simulink model "Experiment1"  (R2025b)
settings: Solver=ode4  StartTime=0.0  StopTime=tsim  FixedStep=baseRate  RelTol=1e-6  AbsTol=1e-6
values from neighbouring files (symbols this model uses):
  a1 = 0.1933    [fmincon_solver_v50.m]    (also in fmincon_solver_v51.m; fmincon_solver_v65_ultrafast.m)
  a2 = 0.1933    [fmincon_solver_v50.m]    (also in fmincon_solver_v51.m; fmincon_solver_v65_ultrafast.m)
  a3 = 0.0621    [fmincon_solver_v50.m]    (also in fmincon_solver_v51.m; fmincon_solver_v65_ultrafast.m)
  b0 = 0.2304    [fmincon_solver_v50.m]    (also in fmincon_solver_v51.m; fmincon_solver_v65_ultrafast.m)
  b1 = 0.1117    [fmincon_solver_v50.m]    (also in fmincon_solver_v51.m; fmincon_solver_v65_ultrafast.m)
  b2 = 0.1057    [fmincon_solver_v50.m]    (also in fmincon_solver_v51.m; fmincon_solver_v65_ultrafast.m)
  b3 = 0.0159    [fmincon_solver_v50.m]    (also in fmincon_solver_v51.m; fmincon_solver_v65_ultrafast.m)
  Gamma1_el = 0.12    [Run_Initializer.m]
  Gamma1_sh = 0.005    [Run_Initializer.m]
  Gamma1_wr = 0.025    [Run_Initializer.m]
  Gamma2_el = 5    [Run_Initializer.m]
  Gamma2_sh = 5    [Run_Initializer.m]
  Gamma2_wr = 5    [Run_Initializer.m]
  Gamma3_el = 10    [Run_Initializer.m]
  Gamma3_sh = 40    [Run_Initializer.m]
  Gamma3_wr = 40    [Run_Initializer.m]
  Gamma4_el = 0.039    [Run_Initializer.m]
  Gamma4_sh = 0.015    [Run_Initializer.m]
  Gamma4_wr = 0.029    [Run_Initializer.m]
  Gamma5_el = 800    [Run_Initializer.m]
  Gamma5_sh = 800    [Run_Initializer.m]
  Gamma5_wr = 800    [Run_Initializer.m]
  Gamma6_el = 0.000001    (= 1e-06)    [Run_Initializer.m]
  Gamma6_sh = 0.005    [Run_Initializer.m]
  Gamma6_wr = 0.02    [Run_Initializer.m]
  Kd_elarm = 0.8    [Run_Initializer.m]
  Kd_sharm = 1.0    (= 1)    [Run_Initializer.m]
  Kd_wrarm = 0.6    [Run_Initializer.m]
  Kp_elarm = 1.2    [Run_Initializer.m]
  Kp_sharm = 1.5    [Run_Initializer.m]
  Kp_wrarm = 1.0    (= 1)    [Run_Initializer.m]
  PWMFreq = 5    [Run_Initializer.m]
  Tz_lim_elarm = .1    (= 0.1)    [Run_Initializer.m]
  Tz_lim_sharm = .1    (= 0.1)    [Run_Initializer.m]
  Tz_lim_wrarm = .1    (= 0.1)    [Run_Initializer.m]
undefined symbols (not defined in the file or in its folder): baseRate, dataRate, DiscIntNeverNeededParam, drop_states_ARM, drop_states_BLACK, drop_states_BLUE, drop_states_RED, F_red_X_nominal, F_red_Y_nominal, F_thrusters_BLACK, F_thrusters_BLUE, F_thrusters_RED, home_states_BLACK, home_states_BLUE, home_states_RED, IBLACK, IBLUE, IDIST, IEE, init_states_BLACK, init_states_BLUE, init_states_RED, IPROX, IRED, K_BLACK, K_BLUE, K_RED, Kd_tb, Kd_tblue, Kd_tr, Kd_xb, Kd_xblue, Kd_xr, Kd_yb, Kd_yblue, Kd_yr, Kp_tb, Kp_tblue, Kp_tr, Kp_xb, Kp_xblue, Kp_xr, Kp_yb, Kp_yblue, Kp_yr, mBLACK, mBLUE, mDIST, mEE, mPROX, mRED, Phase0_End, Phase1_End, Phase2_End, Phase3_End, Phase3_SubPhase1_End, Phase3_SubPhase2_End, Phase3_SubPhase3_End, Phase3_SubPhase4_End, Phase4_End ... (+10)
libraries: simulink x30, nvidiaSharedBlocks x19, MainLibrary x6, dspinverses x3, nvidiaIMUSensorslib x1
(part 7 of 8)

== system Experiment1/Simulate Plant Dynamics/RED and ARM Dynamics/RED + ARM/Calculated & Store Measured States/Subsystem3/Enabled Subsystem ==
  y : Inport
  dt : Inport  Port=2
  Enable : EnablePort
  Constant2 : Constant  Value=0.1
  Delay : Delay  DelayLength=1
  MATLAB Function : MATLAB Function  TreatAsAtomicUnit=on
  dy/dt : Outport
  wires:
  Constant2/1 -> MATLAB Function/3(tau)
  dt/1 -> MATLAB Function/2(dt)
  Delay/1 -> MATLAB Function/4(ema_prev)
  MATLAB Function/2(ema) -> Delay/1
  y/1 -> MATLAB Function/1(y)
  MATLAB Function/1(dy) -> dy/dt/1

== system Experiment1/Simulate Plant Dynamics/RED and ARM Dynamics/RED + ARM/Calculated & Store Measured States/Subsystem4/Enabled Subsystem ==
  y : Inport
  dt : Inport  Port=2
  Enable : EnablePort
  Constant2 : Constant  Value=0.1
  Delay : Delay  DelayLength=1
  MATLAB Function : MATLAB Function  TreatAsAtomicUnit=on
  dy/dt : Outport
  wires:
  Constant2/1 -> MATLAB Function/3(tau)
  dt/1 -> MATLAB Function/2(dt)
  Delay/1 -> MATLAB Function/4(ema_prev)
  MATLAB Function/2(ema) -> Delay/1
  y/1 -> MATLAB Function/1(y)
  MATLAB Function/1(dy) -> dy/dt/1

== system Experiment1/Simulate Plant Dynamics/RED and ARM Dynamics/RED + ARM/Calculated & Store Measured States/Subsystem5/Enabled Subsystem ==
  y : Inport
  dt : Inport  Port=2
  Enable : EnablePort
  Constant2 : Constant  Value=0.1
  Delay : Delay  DelayLength=1
  MATLAB Function : MATLAB Function  TreatAsAtomicUnit=on
  dy/dt : Outport
  wires:
  Constant2/1 -> MATLAB Function/3(tau)
  dt/1 -> MATLAB Function/2(dt)
  Delay/1 -> MATLAB Function/4(ema_prev)
  MATLAB Function/2(ema) -> Delay/1
  y/1 -> MATLAB Function/1(y)
  MATLAB Function/1(dy) -> dy/dt/1

== system Experiment1/Simulate Plant Dynamics/RED and ARM Dynamics/RED + ARM/Data @ Measurement Rate/Calculate True Time Step/Enabled Subsystem3 ==
  y2-y1 : Inport
  Enable : EnablePort
  dy(t)/dt : Outport
  wires:
  y2-y1/1 -> dy(t)/dt/1

== system Experiment1/Simulate Plant Dynamics/RED and ARM Dynamics/RED Only/Calculated & Store Measured States/Subsystem1/Enabled Subsystem ==
  y : Inport
  dt : Inport  Port=2
  Enable : EnablePort
  Constant2 : Constant  Value=0.1
  Delay : Delay  DelayLength=1
  MATLAB Function : MATLAB Function  TreatAsAtomicUnit=on
  dy/dt : Outport
  wires:
  Constant2/1 -> MATLAB Function/3(tau)
  dt/1 -> MATLAB Function/2(dt)
  Delay/1 -> MATLAB Function/4(ema_prev)
  MATLAB Function/2(ema) -> Delay/1
  y/1 -> MATLAB Function/1(y)
  MATLAB Function/1(dy) -> dy/dt/1

== system Experiment1/Simulate Plant Dynamics/RED and ARM Dynamics/RED Only/Calculated & Store Measured States/Subsystem2/Enabled Subsystem ==
  y : Inport
  dt : Inport  Port=2
  Enable : EnablePort
  Constant2 : Constant  Value=0.1
  Delay : Delay  DelayLength=1
  MATLAB Function : MATLAB Function  TreatAsAtomicUnit=on
  dy/dt : Outport
  wires:
  Constant2/1 -> MATLAB Function/3(tau)
  dt/1 -> MATLAB Function/2(dt)
  Delay/1 -> MATLAB Function/4(ema_prev)
  MATLAB Function/2(ema) -> Delay/1
  y/1 -> MATLAB Function/1(y)
  MATLAB Function/1(dy) -> dy/dt/1

== system Experiment1/Simulate Plant Dynamics/RED and ARM Dynamics/RED Only/Data @ Measurement Rate/Calculate True Time Step/Enabled Subsystem3 ==
  y2-y1 : Inport
  Enable : EnablePort
  dy(t)/dt : Outport
  wires:
  y2-y1/1 -> dy(t)/dt/1

== matlab function Experiment1/3 - Control/Default LQR Control (BLUE)/Calculate Error/MATLAB Function ==
  data: Rz_path input; Rz_error output; Rz_measured input
function Rz_error = SmoothAngularDifference(Rz_path, Rz_measured)

    Rz_error = mod(Rz_measured-Rz_path+pi, 2*pi)-pi;


end

== matlab function Experiment1/3 - Control/Default PD Control (BLUE)/Calculate Error/MATLAB Function ==
  data: Rz_path input; Rz_error output; Rz_measured input
function Rz_error = SmoothAngularDifference(Rz_path, Rz_measured)

    Rz_error = mod(Rz_measured-Rz_path+pi, 2*pi)-pi;


end

== matlab function Experiment1/Simulate Plant Dynamics/RED and ARM Dynamics/RED + ARM/Calculated & Store Measured States/Subsystem3/Enabled Subsystem/MATLAB Function ==
  data: y input; dy output; dt input; tau input; ema_prev input; ema output
function [dy, ema] = realtime_derivative_ema(y, dt, tau, ema_prev)
    % Compute smoothed derivative using Exponential Moving Average
    %
    % Inputs:
    %   y        : Current measurement
    %   dt       : Time step
    %   tau      : Time constant for EMA filter (larger = more smoothing)
    %   ema_prev : Previous EMA value
    %
    % Outputs:
    %   dy  : Smoothed derivative estimate
    %   ema : Updated EMA value
    
    % Calculate smoothing factor from time constant
    alpha = 1 - exp(-dt ./ tau);
    
    % Update Exponential Moving Average
    ema = alpha .* y + (1 - alpha) .* ema_prev;
    
    % Compute derivative using finite difference on smoothed values
    dy = (ema - ema_prev) ./ dt;
end

== matlab function Experiment1/Simulate Plant Dynamics/RED and ARM Dynamics/RED Only/Calculated & Store Measured States/Subsystem2/Enabled Subsystem/MATLAB Function ==
  data: y input; dy output; dt input; tau input; ema_prev input; ema output
function [dy, ema] = realtime_derivative_ema(y, dt, tau, ema_prev)
    % Compute smoothed derivative using Exponential Moving Average
    %
    % Inputs:
    %   y        : Current measurement
    %   dt       : Time step
    %   tau      : Time constant for EMA filter (larger = more smoothing)
    %   ema_prev : Previous EMA value
    %
    % Outputs:
    %   dy  : Smoothed derivative estimate
    %   ema : Updated EMA value
    
    % Calculate smoothing factor from time constant
    alpha = 1 - exp(-dt ./ tau);
    
    % Update Exponential Moving Average
    ema = alpha .* y + (1 - alpha) .* ema_prev;
    
    % Compute derivative using finite difference on smoothed values
    dy = (ema - ema_prev) ./ dt;
end

== matlab function Experiment1/Simulate Plant Dynamics/BLACK Dynamics/Calculated & Store Measured States/Subsystem1/Enabled Subsystem/MATLAB Function ==
  data: y input; dy output; dt input; tau input; ema_prev input; ema output
function [dy, ema] = realtime_derivative_ema(y, dt, tau, ema_prev)
    % Compute smoothed derivative using Exponential Moving Average
    %
    % Inputs:
    %   y        : Current measurement
    %   dt       : Time step
    %   tau      : Time constant for EMA filter (larger = more smoothing)
    %   ema_prev : Previous EMA value
    %
    % Outputs:
    %   dy  : Smoothed derivative estimate
    %   ema : Updated EMA value
    
    % Calculate smoothing factor from time constant
    alpha = 1 - exp(-dt ./ tau);
    
    % Update Exponential Moving Average
    ema = alpha .* y + (1 - alpha) .* ema_prev;
    
    % Compute derivative using finite difference on smoothed values
    dy = (ema - ema_prev) ./ dt;
end

== matlab function Experiment1/Simulate Plant Dynamics/RED and ARM Dynamics/RED Only/Data @ Measurement Rate/Calculate True Time Step/MATLAB Function ==
  data: dt input; dt_out output; dataRate input
function dt_out = CheckforInvalidTime(dt, dataRate)

    if dt <= 0

        dt_out = dataRate;

    else

        dt_out = dt;

    end


end

== matlab function Experiment1/Thruster Control Code/Change BLACK Behavior/Calculate Duty Cycle/MATLAB Function5 ==
  data: H_final output; u_desired input; duty_cycles output; x0 input; thruster_dist2CG_RED parameter; F_red_X_nominal parameter; F_red_Y_nominal parameter; max_iters parameter; tol parameter
function [H_final, duty_cycles] = optimize_duty_cycle_with_decay( ...
    u_desired, x0, thruster_dist2CG_RED, F_red_X_nominal, F_red_Y_nominal, max_iters, tol)
    %OPTIMIZE_DUTY_CYCLE_WITH_DECAY 
    %   Iteratively optimizes thruster duty cycles while updating thrust decay.
    %
    %   Inputs:
    %       u_desired           - Desired force/torque vector [Fx; Fy; M] (3x1)
    %       x0                  - Initial guess for duty cycles (8x1)
    %       thruster_dist2CG_RED- Distances of thrusters from CG (vector, mm)
    %       F_red_X_nominal     - Nominal X-direction thruster force (scalar, N)
    %       F_red_Y_nominal     - Nominal Y-direction thruster force (scalar, N)
    %       max_iters           - Maximum optimization iterations
    %       tol                 - Convergence tolerance (on duty cycles)
    %
    %   Outputs:
    %       H_final     - Final H-matrix including thrust decay (3x8)
    %       duty_cycles - Optimized duty cycles (8x1)
    %

    % ---------------------------
    % Initialization
    % ---------------------------
    num_thrusters      = length(x0); %#ok<NASGU> % reserved if needed later
    duty_cycles        = x0;                     % current solution
    thrust_decay_factor = 1;                     % initial decay
    prev_duty_cycles   = duty_cycles + 2*tol;    % force first iteration

    % ---------------------------
    % Iterative optimization
    % ---------------------------
    for iter = 1:max_iters
        % Build system matrix H with current decay factor
        H = MakeHWithDecay(thruster_dist2CG_RED, F_red_X_nominal, ...
                           thrust_decay_factor, F_red_Y_nominal);

        % Solve constrained least squares (box constraints: 0 ≤ x ≤ 1)
        duty_cycles = custom_constrained_least_squares(H, u_desired, duty_cycles);

        % Update decay factor based on the current duty cycles
        [thrust_decay_factor, ~] = check_thrust_decay(duty_cycles);

        % Check convergence (∞-norm difference)
        if norm(duty_cycles - prev_duty_cycles, Inf) < tol
            H_final = MakeHWithDecayRecalculateForce(thruster_dist2CG_RED, ...
                        F_red_X_nominal, thrust_decay_factor, F_red_Y_nominal);
            return;
        end

        % Update reference for next iteration
        prev_duty_cycles = duty_cycles;
    end

    % If not converged within max_iters, return final H with last decay
    H_final = MakeHWithDecayRecalculateForce(thruster_dist2CG_RED, ...
                F_red_X_nominal, thrust_decay_factor, F_red_Y_nominal);
end


% ========================================================================
% Custom Constrained Least Squares Solver
% ========================================================================
function x_opt = custom_constrained_least_squares(H, b, x0)
    %CUSTOM_CONSTRAINED_LEAST_SQUARES
    %   Solves min_x ||H*x - b||^2 subject to 0 <= x <= 1
    %   using projected gradient descent with backtracking line search.
    %
    %   Inputs:
    %       H   - System matrix (3x8)
    %       b   - Desired vector (3x1)
    %       x0  - Initial guess (8x1)
    %
    %   Output:
    %       x_opt - Optimal duty cycle vector (8x1)

    % Parameters
    max_iterations = 100;
    tolerance      = 1e-6;
    alpha          = 0.01;  % initial step size
    beta           = 0.5;   % backtracking factor

    % Initialization
    x      = x0;
    x_prev = x0 + 2*tolerance;

    % Precompute matrices
    HtH = H' * H;
    Htb = H' * b;

    for iter = 1:max_iterations
        % Gradient of ||H*x - b||^2
        gradient = 2 * (HtH*x - Htb);

        % Store objective for comparison
        current_obj = norm(H*x - b)^2;

        % Backtracking line search
        step_size = alpha;
        for ls_iter = 1:20
            x_new = x - step_size * gradient;
            x_new = max(0, min(1, x_new)); % project into [0,1]

            new_obj = norm(H*x_new - b)^2;
            if new_obj < current_obj
                break; % accept step
            else
                step_size = step_size * beta;
            end
        end

        % Update
        x = x_new;

        % Convergence check
        if norm(x - x_prev) < tolerance
            break;
        end

        % Adaptive step size tuning
        if iter > 1 && new_obj < current_obj
            alpha = min(alpha * 1.1, 0.1); % speed up if progress
        else
            alpha = alpha * 0.9;           % slow down otherwise
        end

        % Store for next iteration
        x_prev = x;
    end

    x_opt = x;
end


% ========================================================================
% Construct H-matrix (with decay factor)
% ========================================================================
function H = MakeHWithDecay(thruster_dist2CG, F_X_nominal, thrust_decay_factor, F_Y_nominal)
    %MAKEHWITHDECAY
    %   Builds the H matrix that maps thruster duty cycles to [Fx; Fy; M],
    %   applying thrust decay.
    %
    %   Outputs H as (3x8)

    % Convert thruster arm distances to meters
    adjusted_dist = thruster_dist2CG / 1000;

    % Thruster directions (X, Y, and moment arm)
    Vec1 = [-1; -1;  0;  0;  1;  1;  0;  0]; % X
    Vec2 = [ 0;  0;  1;  1;  0;  0; -1; -1]; % Y
    Vec3 = adjusted_dist;                    % moment (Z)

    Mat1 = [Vec1, Vec2, Vec3]';

    % Thruster forces (scaled by decay)
    F_thrusters = [F_X_nominal; F_X_nominal; ...
                   F_Y_nominal; F_Y_nominal; ...
                   F_X_nominal; F_X_nominal; ...
                   F_Y_nominal; F_Y_nominal] * thrust_decay_factor;

    % Build diagonal scaling
    Mat2 = diag(F_thrusters / 2);

    % Final mapping
    H = Mat1 * Mat2;
end


% ========================================================================
% Construct H-matrix (recalculate full force with decay)
% ========================================================================
function H = MakeHWithDecayRecalculateForce(thruster_dist2CG, F_X_nominal, thrust_decay_factor, F_Y_nominal)
    %MAKEHWITHDECAYRECALCULATEFORCE
    %   Same as MakeHWithDecay but applies full nominal force scaling.

    adjusted_dist = thruster_dist2CG / 1000;

    Vec1 = [-1; -1;  0;  0;  1;  1;  0;  0];
    Vec2 = [ 0;  0;  1;  1;  0;  0; -1; -1];
    Vec3 = adjusted_dist;

    Mat1 = [Vec1, Vec2, Vec3]';

    F_thrusters = [F_X_nominal; F_X_nominal; ...
                   F_Y_nominal; F_Y_nominal; ...
                   F_X_nominal; F_X_nominal; ...
                   F_Y_nominal; F_Y_nominal] * thrust_decay_factor;

    Mat2 = diag(F_thrusters);

    H = Mat1 * Mat2;
end


% ========================================================================
% Thrust Decay Update Rule
% ========================================================================
function [thrust_decay_factor, count] = check_thrust_decay(PWMs)
    %CHECK_THRUST_DECAY
    %   Updates thrust decay factor based on average duty cycle.
    %
    %   Inputs:
    %       PWMs - Duty cycle vector (8x1)
    %
    %   Outputs:
    %       thrust_decay_factor - Adjusted decay factor (scalar)
    %       count               - Number of active thrusters

    % Normalize if needed
    if max(PWMs) > 1
        PWMs = PWMs / max(PWMs);
    end
    
    % Active thrusters
    count = sum(PWMs > 0);
    
    % Mean duty cycle (only active thrusters)
    avg_duty = sum(max(PWMs, 0)) / max(count, 1);
    
    % Update rule (piecewise)
    if avg_duty < 0.3 || count == 0
        thrust_decay_factor = 1;
    else
        thrust_decay_factor = max(0.6 - 2*avg_duty + 1, 0.5);
    end
end

== matlab function Experiment1/Simulate Plant Dynamics/RED and ARM Dynamics/RED + ARM/Calculated & Store Measured States/Subsystem4/Enabled Subsystem/MATLAB Function ==
  data: y input; dy output; dt input; tau input; ema_prev input; ema output
function [dy, ema] = realtime_derivative_ema(y, dt, tau, ema_prev)
    % Compute smoothed derivative using Exponential Moving Average
    %
    % Inputs:
    %   y        : Current measurement
    %   dt       : Time step
    %   tau      : Time constant for EMA filter (larger = more smoothing)
    %   ema_prev : Previous EMA value
    %
    % Outputs:
    %   dy  : Smoothed derivative estimate
    %   ema : Updated EMA value
    
    % Calculate smoothing factor from time constant
    alpha = 1 - exp(-dt ./ tau);
    
    % Update Exponential Moving Average
    ema = alpha .* y + (1 - alpha) .* ema_prev;
    
    % Compute derivative using finite difference on smoothed values
    dy = (ema - ema_prev) ./ dt;
end

== matlab function Experiment1/PhaseSpace Camera Code/Use Hardware to Obtain States/Store RED Data/Subsystem1/Enabled Subsystem/MATLAB Function ==
  data: y input; dy output; dt input; tau input; ema_prev input; ema output
function [dy, ema] = realtime_derivative_ema(y, dt, tau, ema_prev)
    % Compute smoothed derivative using Exponential Moving Average
    %
    % Inputs:
    %   y        : Current measurement
    %   dt       : Time step
    %   tau      : Time constant for EMA filter (larger = more smoothing)
    %   ema_prev : Previous EMA value
    %
    % Outputs:
    %   dy  : Smoothed derivative estimate
    %   ema : Updated EMA value
    
    % Calculate smoothing factor from time constant
    alpha = 1 - exp(-dt ./ tau);
    
    % Update Exponential Moving Average
    ema = alpha .* y + (1 - alpha) .* ema_prev;
    
    % Compute derivative using finite difference on smoothed values
    dy = (ema - ema_prev) ./ dt;
end

== matlab function Experiment1/Simulate Plant Dynamics/BLACK Dynamics/Calculated & Store Measured States/Subsystem2/Enabled Subsystem/MATLAB Function ==
  data: y input; dy output; dt input; tau input; ema_prev input; ema output
function [dy, ema] = realtime_derivative_ema(y, dt, tau, ema_prev)
    % Compute smoothed derivative using Exponential Moving Average
    %
    % Inputs:
    %   y        : Current measurement
    %   dt       : Time step
    %   tau      : Time constant for EMA filter (larger = more smoothing)
    %   ema_prev : Previous EMA value
    %
    % Outputs:
    %   dy  : Smoothed derivative estimate
    %   ema : Updated EMA value
    
    % Calculate smoothing factor from time constant
    alpha = 1 - exp(-dt ./ tau);
    
    % Update Exponential Moving Average
    ema = alpha .* y + (1 - alpha) .* ema_prev;
    
    % Compute derivative using finite difference on smoothed values
    dy = (ema - ema_prev) ./ dt;
end

== matlab function Experiment1/Simulate Plant Dynamics/RED and ARM Dynamics/RED + ARM/Coriolis Function1 ==
  data: a1 parameter; a2 parameter; a3 parameter; b0 parameter; b1 parameter; b2 parameter; mPROX parameter; mDIST parameter; mEE parameter; Phi parameter; CoriolisS output; x input
function CoriolisS = CoriolisFunc3LINK(a1,a2,a3,b0,b1,b2,mPROX,mDIST,mEE,Phi,x)
%CORIOLISFUNC3LINK
%    CORIOLISS = CORIOLISFUNC3LINK(A1,A2,A3,B0,B1,B2,mPROX,mDIST,mEE,PHI,Q0,Q1,Q2,Q3,Q0_DOT,Q1_DOT,Q2_DOT,Q3_DOT)

%    This function was generated by the Symbolic Math Toolbox version 8.0.
%    05-Nov-2017 11:48:44

q0 = x(3);
q1 = x(4);
q2 = x(5);
q3 = x(6);

q0_dot = x(9);
q1_dot = x(10);
q2_dot = x(11);
q3_dot = x(12);

t2 = a1+b1;
t3 = a1.*mPROX;
t4 = mDIST.*t2;
t5 = mEE.*t2;
t6 = t3+t4+t5;
t7 = a2.*mDIST;
t8 = a2+b2;
t9 = mEE.*t8;
t10 = t7+t9;
t11 = pi.*(1.0./2.0);
t12 = q0_dot.*t6;
t13 = q1_dot.*t6;
t14 = q0+q1+t11;
t15 = cos(t14);
t16 = t12+t13;
t17 = q0_dot.*t10;
t18 = q1_dot.*t10;
t19 = q2_dot.*t10;
t20 = q0+q1+q2+t11;
t21 = cos(t20);
t22 = t17+t18+t19;
t23 = a3.*mEE.*q0_dot;
t24 = a3.*mEE.*q1_dot;
t25 = a3.*mEE.*q2_dot;
t26 = a3.*mEE.*q3_dot;
t27 = q0+q1+q2+q3+t11;
t28 = cos(t27);
t29 = t23+t24+t25+t26;
t30 = b0.*mPROX;
t31 = b0.*mDIST;
t32 = b0.*mEE;
t33 = t30+t31+t32;
t34 = (pi/2-Phi)+q0;
t35 = sin(t14);
t36 = sin(t20);
t37 = sin(t27);
t38 = q0_dot+q1_dot+q2_dot+q3_dot;
t39 = q0+q1+q2+q3;
t40 = a1.*b0.*mPROX.*q1_dot;
t41 = a1.*b0.*mDIST.*q1_dot;
t42 = a1.*b0.*mEE.*q1_dot;
t43 = b0.*b1.*mDIST.*q1_dot;
t44 = b0.*b1.*mEE.*q1_dot;
t45 = (pi/2-Phi)-q1;
t46 = cos(t45);
t47 = a2.*b0.*mDIST.*q1_dot;
t48 = a2.*b0.*mDIST.*q2_dot;
t49 = a2.*b0.*mEE.*q1_dot;
t50 = a2.*b0.*mEE.*q2_dot;
t51 = b0.*b2.*mEE.*q1_dot;
t52 = b0.*b2.*mEE.*q2_dot;
t53 = -(pi/2-Phi)+q1+q2;
t54 = cos(t53);
t55 = a3.*b0.*mEE.*q1_dot;
t56 = a3.*b0.*mEE.*q2_dot;
t57 = a3.*b0.*mEE.*q3_dot;
t58 = -(pi/2-Phi)+q1+q2+q3;
t59 = cos(t58);
t60 = a2.*b1.*mDIST.*q2_dot;
t61 = a1.*b2.*mEE.*q2_dot;
t62 = a2.*b1.*mEE.*q2_dot;
t63 = b1.*b2.*mEE.*q2_dot;
t64 = a1.*a2.*mDIST.*q2_dot;
t65 = a1.*a2.*mEE.*q2_dot;
t66 = sin(q2);
t67 = t60+t61+t62+t63+t64+t65;
t68 = a3.*b2.*mEE.*q3_dot;
t69 = a2.*a3.*mEE.*q3_dot;
t70 = sin(q3);
t71 = t68+t69;
t72 = a3.*b1.*mEE.*q2_dot;
t73 = a3.*b1.*mEE.*q3_dot;
t74 = a1.*a3.*mEE.*q2_dot;
t75 = a1.*a3.*mEE.*q3_dot;
t76 = q2+q3;
t77 = sin(t76);
t78 = t72+t73+t74+t75;
t79 = a2.*b0.*mDIST.*q0_dot;
t80 = a2.*b0.*mEE.*q0_dot;
t81 = b0.*b2.*mEE.*q0_dot;
t82 = t47+t48+t49+t50+t51+t52+t79+t80+t81;
t83 = a3.*b0.*mEE.*q0_dot;
t84 = t55+t56+t57+t83;
t85 = a1.*b0.*mPROX.*q0_dot;
t86 = a1.*b0.*mDIST.*q0_dot;
t87 = a1.*b0.*mEE.*q0_dot;
t88 = b0.*b1.*mDIST.*q0_dot;
t89 = b0.*b1.*mEE.*q0_dot;
t90 = a2.*b1.*mDIST.*q0_dot;
t91 = a1.*b2.*mEE.*q0_dot;
t92 = a2.*b1.*mDIST.*q1_dot;
t93 = a2.*b1.*mEE.*q0_dot;
t94 = a1.*b2.*mEE.*q1_dot;
t95 = a2.*b1.*mEE.*q1_dot;
t96 = b1.*b2.*mEE.*q0_dot;
t97 = b1.*b2.*mEE.*q1_dot;
t98 = a1.*a2.*mDIST.*q0_dot;
t99 = a1.*a2.*mDIST.*q1_dot;
t100 = a1.*a2.*mEE.*q0_dot;
t101 = a1.*a2.*mEE.*q1_dot;
t102 = t60+t61+t62+t63+t64+t65+t90+t91+t92+t93+t94+t95+t96+t97+t98+t99+t100+t101;
t103 = a3.*b1.*mEE.*q0_dot;
t104 = a3.*b1.*mEE.*q1_dot;
t105 = a1.*a3.*mEE.*q0_dot;
t106 = a1.*a3.*mEE.*q1_dot;
t107 = t72+t73+t74+t75+t103+t104+t105+t106;
t108 = t79+t80+t81;
t109 = t54.*t108;
t110 = t59.*t83;
t111 = t90+t91+t92+t93+t94+t95+t96+t97+t98+t99+t100+t101;
t112 = t66.*t111;
t113 = t103+t104+t105+t106;
t114 = t77.*t113;
t115 = a2.*q0_dot;
t116 = a2.*q1_dot;
t117 = a2.*q2_dot;
t118 = b2.*q0_dot;
t119 = b2.*q1_dot;
t120 = b2.*q2_dot;
t121 = t115+t116+t117+t118+t119+t120;
t122 = a3.*mEE.*t70.*t121;
t123 = a1.*q0_dot;
t124 = a1.*q1_dot;
t125 = b1.*q0_dot;
t126 = b1.*q1_dot;
t127 = t123+t124+t125+t126;
t128 = a3.*mEE.*t77.*t127;
CoriolisS = reshape([0.0,0.0,0.0,0.0,0.0,0.0,0.0,0.0,0.0,0.0,0.0,0.0,-t15.*t16-t21.*t22-t28.*t29-q0_dot.*t33.*cos(t34),-t16.*t35-t22.*t36-t29.*t37-q0_dot.*t33.*sin(t34),-t66.*t67-t70.*t71-t77.*t78-t46.*(t40+t41+t42+t43+t44)-t59.*(t55+t56+t57)-t54.*(t47+t48+t49+t50+t51+t52),t109+t110-t66.*t67-t70.*t71-t77.*t78+t46.*(t85+t86+t87+t88+t89),t109+t110+t112+t114-t70.*t71,t110+t122+t128,-t15.*t16-t21.*t22-t28.*t29,-t16.*t35-t22.*t36-t29.*t37,-t66.*t67-t54.*t82-t70.*t71-t59.*t84-t77.*t78-t46.*(t40+t41+t42+t43+t44+t85+t86+t87+t88+t89),-t66.*t67-t70.*t71-t77.*t78,t112+t114-t70.*t71,t122+t128,-t21.*t22-t28.*t29,-t22.*t36-t29.*t37,-t54.*t82-t70.*t71-t59.*t84-t66.*t102-t77.*t107,-t70.*t71-t66.*t102-t77.*t107,-a3.*mEE.*q3_dot.*t8.*t70,a3.*mEE.*t8.*t70.*(q0_dot+q1_dot+q2_dot),a3.*mEE.*t38.*sin(t39),-a3.*mEE.*t38.*cos(t39),-a3.*b0.*mEE.*t38.*t59-a3.*mEE.*t8.*t38.*t70-a3.*mEE.*t2.*t38.*t77,-a3.*mEE.*t8.*t38.*t70-a3.*mEE.*t2.*t38.*t77,-a3.*mEE.*t8.*t38.*t70,0.0],[6,6]);
end

== matlab function Experiment1/Simulate Plant Dynamics/BLACK Dynamics/Data @ Measurement Rate/Calculate True Time Step/MATLAB Function ==
  data: dt input; dt_out output; dataRate input
function dt_out = CheckforInvalidTime(dt, dataRate)

    if dt <= 0

        dt_out = dataRate;

    else

        dt_out = dt;

    end


end

== matlab function Experiment1/Simulate Plant Dynamics/RED and ARM Dynamics/RED + ARM/Inertia Function 1 ==
  data: mRED parameter; IRED parameter; Phi parameter; b0 parameter; a1 parameter; b1 parameter; a2 parameter; b2 parameter; a3 parameter; b3 parameter; mPROX parameter; mDIST parameter; mEE parameter; IPROX parameter; IDIST parameter; InertiaS output; x input; IEE parameter
function InertiaS = InertiaFunc3LINK(mRED, IRED, Phi, b0, a1, b1, a2, b2, a3, b3, mPROX, mDIST, mEE, IPROX, IDIST, x, IEE)

    q0 = x(3);
    q1 = x(4);
    q2 = x(5);
    q3 = x(6);
    
    t2 = a1+b1;
    t3 = a1.*mPROX;
    t4 = mDIST.*t2;
    t5 = mEE.*t2;
    t6 = q0+q1;
    t7 = cos(t6);
    t8 = t3+t4+t5;
    t9 = a2.*mDIST;
    t10 = a2+b2;
    t11 = mEE.*t10;
    t12 = q0+q1+q2;
    t13 = cos(t12);
    t14 = t9+t11;
    t15 = q0+q1+q2+q3;
    t16 = cos(t15);
    t17 = mRED+mPROX+mDIST+mEE;
    t18 = b0.*mPROX;
    t19 = b0.*mDIST;
    t20 = b0.*mEE;
    t21 = t18+t19+t20;
    t22 = (pi/2-Phi)+q0;
    t23 = sin(t6);
    t24 = sin(t12);
    t25 = sin(t15);
    t26 = a2.*mEE;
    t27 = b2.*mEE;
    t28 = t9+t26+t27;
    t29 = sin(t22);
    t86 = t7.*t8;
    t87 = t13.*t14;
    t88 = a3.*mEE.*t16;
    t30 = -t86-t87-t88-t21.*t29;
    t31 = cos(t22);
    t32 = t21.*t31;
    t89 = t8.*t23;
    t90 = t14.*t24;
    t91 = a3.*mEE.*t25;
    t33 = t32-t89-t90-t91;
    t34 = a1.^2;
    t35 = a2.^2;
    t36 = b0.^2;
    t37 = b1.^2;
    t38 = a1.*a2.*mDIST.*2.0;
    t39 = a1.*a2.*mEE.*2.0;
    t40 = a2.*b1.*mDIST.*2.0;
    t41 = a1.*b2.*mEE.*2.0;
    t42 = a2.*b1.*mEE.*2.0;
    t43 = b1.*b2.*mEE.*2.0;
    t44 = t38+t39+t40+t41+t42+t43;
    t45 = cos(q2);
    t46 = t44.*t45;
    t47 = a2.*a3.*mEE.*2.0;
    t48 = a3.*b2.*mEE.*2.0;
    t49 = t47+t48;
    t50 = cos(q3);
    t51 = t49.*t50;
    t52 = a1.*a3.*mEE.*2.0;
    t53 = a3.*b1.*mEE.*2.0;
    t54 = t52+t53;
    t55 = q2+q3;
    t56 = cos(t55);
    t57 = t54.*t56;
    t58 = (pi/2-Phi)-q1;
    t59 = sin(t58);
    t60 = -(pi/2-Phi)+q1+q2;
    t61 = sin(t60);
    t62 = -(pi/2-Phi)+q1+q2+q3;
    t63 = sin(t62);
    t64 = mPROX.*t34;
    t65 = mDIST.*t34;
    t66 = mEE.*t34;
    t67 = mDIST.*t35;
    t68 = mEE.*t35;
    t69 = a3.^2;
    t70 = mEE.*t69;
    t71 = mDIST.*t37;
    t72 = mEE.*t37;
    t73 = b2.^2;
    t74 = mEE.*t73;
    t75 = a1.*b1.*mDIST.*2.0;
    t76 = a1.*b1.*mEE.*2.0;
    t77 = a2.*b2.*mEE.*2.0;
    t78 = a2.*b0.*mDIST;
    t79 = a2.*b0.*mEE;
    t80 = b0.*b2.*mEE;
    t81 = t78+t79+t80;
    t82 = a1.*a3.*mEE;
    t83 = a3.*b1.*mEE;
    t84 = t82+t83;
    t85 = t56.*t84;
    t92 = a1.*b0.*mPROX;
    t93 = a1.*b0.*mDIST;
    t94 = a1.*b0.*mEE;
    t95 = b0.*b1.*mDIST;
    t96 = b0.*b1.*mEE;
    t97 = t92+t93+t94+t95+t96;
    t98 = t59.*t97;
    t112 = t61.*t81;
    t113 = a3.*b0.*mEE.*t63;
    t99 = IPROX+IDIST+IEE+t46+t51+t57+t64+t65+t66+t67+t68+t70+t71+t72+t74+t75+t76+t77+t98-t112-t113;
    t100 = a1.*a2.*mDIST;
    t101 = a1.*a2.*mEE;
    t102 = a2.*b1.*mDIST;
    t103 = a1.*b2.*mEE;
    t104 = a2.*b1.*mEE;
    t105 = b1.*b2.*mEE;
    t106 = t100+t101+t102+t103+t104+t105;
    t107 = t45.*t106;
    t108 = a2.*a3.*mEE;
    t109 = a3.*b2.*mEE;
    t110 = t108+t109;
    t111 = t50.*t110;
    t114 = IDIST+IEE+t51+t67+t68+t70+t74+t77+t85+t107;
    t115 = IEE+t70+t85+t111;
    t116 = IEE+t70+t111;
    InertiaS = reshape([t17,0.0,t30,-t86-t87-t88,-t88-t13.*t28,-t88,0.0,t17,t33,-t89-t90-t91,-t91-t24.*t28,-t91,t30,t33,IRED+IPROX+IDIST+IEE+t46+t51+t57+t64+t65+t66+t67+t68+t70+t71+t72+t74+t75+t76+t77+t59.*(a1.*b0.*mPROX.*2.0+a1.*b0.*mDIST.*2.0+a1.*b0.*mEE.*2.0+b0.*b1.*mDIST.*2.0+b0.*b1.*mEE.*2.0)+mPROX.*t36+mDIST.*t36+mEE.*t36-t61.*(a2.*b0.*mDIST.*2.0+a2.*b0.*mEE.*2.0+b0.*b2.*mEE.*2.0)-a3.*b0.*mEE.*t63.*2.0,t99,IDIST+IEE+t51+t67+t68+t70+t74+t77+t85+t107-t112-t113,IEE+t70+t85+t111-t113,-t7.*t8-t13.*t14-a3.*mEE.*t16,-t8.*t23-t14.*t24-a3.*mEE.*t25,t99,IPROX+IDIST+IEE+t46+t51+t57+t64+t65+t66+t67+t68+t70+t71+t72+t74+t75+t76+t77,t114,t115,-t13.*t28-a3.*mEE.*t16,-t24.*t28-a3.*mEE.*t25,IDIST+IEE+t51+t67+t68+t70+t74+t77+t85+t107-t61.*t81-a3.*b0.*mEE.*t63,t114,IDIST+IEE+t51+t67+t68+t70+t74+t77,t116,-a3.*mEE.*t16,-a3.*mEE.*t25,IEE+t70+t85+t111-a3.*b0.*mEE.*t63,t115,t116,IEE+t70],[6,6]);
end

== matlab function Experiment1/Simulate Plant Dynamics/BLUE Dynamics/Calculated & Store Measured States/Subsystem1/Enabled Subsystem/MATLAB Function ==
  data: y input; dy output; dt input; tau input; ema_prev input; ema output
function [dy, ema] = realtime_derivative_ema(y, dt, tau, ema_prev)
    % Compute smoothed derivative using Exponential Moving Average
    %
    % Inputs:
    %   y        : Current measurement
    %   dt       : Time step
    %   tau      : Time constant for EMA filter (larger = more smoothing)
    %   ema_prev : Previous EMA value
    %
    % Outputs:
    %   dy  : Smoothed derivative estimate
    %   ema : Updated EMA value
    
    % Calculate smoothing factor from time constant
    alpha = 1 - exp(-dt ./ tau);
    
    % Update Exponential Moving Average
    ema = alpha .* y + (1 - alpha) .* ema_prev;
    
    % Compute derivative using finite difference on smoothed values
    dy = (ema - ema_prev) ./ dt;
end

== matlab function Experiment1/Simulate Plant Dynamics/BLACK Dynamics/Dynamics Model for BLACK/MATLAB Function ==
  data: control_inputs input; x_ddot output; mBLACK parameter; IBLACK parameter
function x_ddot = BLACK_dynamics(control_inputs, mBLACK, IBLACK)

%#codegen
% Fully define the size of x_ddot() for code generation:
x_ddot     = zeros(3,1);

% Extract the control inputs from the control_input vector:
Fx        = control_inputs(1);              % [N]
Fy        = control_inputs(2);              % [N]
Tz        = control_inputs(3);              % [N.m]

% Calculate the state acceleration vector:
x_ddot(1) = Fx/mBLACK;                      % [m/s^2]
x_ddot(2) = Fy/mBLACK;                      % [m/s^2]
x_ddot(3) = Tz/IBLACK;                      % [rad/s^2]

end

== matlab function Experiment1/Simulate Plant Dynamics/BLUE Dynamics/BLUE  Dynamics Model/MATLAB Function ==
  data: control_inputs input; x_ddot output; mBLUE parameter; IBLUE parameter
function x_ddot = BLUE_dynamics(control_inputs, mBLUE, IBLUE)%#codegen
% Fully define the size of x_ddot() for code generation:
x_ddot     = zeros(3,1);

% Extract the control inputs from the control_input vector:
Fx        = control_inputs(1);              % [N]
Fy        = control_inputs(2);              % [N]
Tz        = control_inputs(3);              % [N.m]

% Calculate the state acceleration vector:
x_ddot(1) = Fx/mBLUE;                      % [m/s^2]
x_ddot(2) = Fy/mBLUE;                      % [m/s^2]
x_ddot(3) = Tz/IBLUE;                      % [rad/s^2]

end

== matlab function Experiment1/Gyro.//Accel. Code/Log Gyro//Accel/Parse IMU Data ==
  data: WhoAmI input; RED_IMU_Ax output; IMU_Ax input; IMU_Ay input; IMU_Gz input; RED_IMU_Ay output; RED_IMU_Gz output; BLACK_IMU_Ax output; BLACK_IMU_Ay output; BLACK_IMU_Gz output; BLUE_IMU_Ax output; BLUE_IMU_Ay output; BLUE_IMU_Gz output
function [RED_IMU_Ax, RED_IMU_Ay, RED_IMU_Gz, BLACK_IMU_Ax, BLACK_IMU_Ay, BLACK_IMU_Gz, BLUE_IMU_Ax, BLUE_IMU_Ay, BLUE_IMU_Gz] = ParseIMUData(WhoAmI, IMU_Ax, IMU_Ay, IMU_Gz)

    if WhoAmI == 1 % This is RED

        RED_IMU_Ax = IMU_Ax;
        RED_IMU_Ay = IMU_Ay;
        RED_IMU_Gz = IMU_Gz;
        BLACK_IMU_Ax = 0;
        BLACK_IMU_Ay = 0;
        BLACK_IMU_Gz = 0;
        BLUE_IMU_Ax = 0;
        BLUE_IMU_Ay = 0;
        BLUE_IMU_Gz = 0;

    elseif WhoAmI == 2 % This is BLACK

        RED_IMU_Ax = 0;
        RED_IMU_Ay = 0;
        RED_IMU_Gz = 0;
        BLACK_IMU_Ax = IMU_Ax;
        BLACK_IMU_Ay = IMU_Ay;
        BLACK_IMU_Gz = IMU_Gz;
        BLUE_IMU_Ax = 0;
        BLUE_IMU_Ay = 0;
        BLUE_IMU_Gz = 0;

    elseif WhoAmI == 3 % This is BLUE

        RED_IMU_Ax = 0;
        RED_IMU_Ay = 0;
        RED_IMU_Gz = 0;
        BLACK_IMU_Ax = 0;
        BLACK_IMU_Ay = 0;
        BLACK_IMU_Gz = 0;
        BLUE_IMU_Ax = IMU_Ax;
        BLUE_IMU_Ay = IMU_Ay;
        BLUE_IMU_Gz = IMU_Gz;

    else 

        RED_IMU_Ax = 0;
        RED_IMU_Ay = 0;
        RED_IMU_Gz = 0;
        BLACK_IMU_Ax = 0;
        BLACK_IMU_Ay = 0;
        BLACK_IMU_Gz = 0;
        BLUE_IMU_Ax = 0;
        BLUE_IMU_Ay = 0;
        BLUE_IMU_Gz = 0;       

    end

end

== matlab function Experiment1/Simulate Plant Dynamics/BLUE Dynamics/Calculated & Store Measured States/Subsystem2/Enabled Subsystem/MATLAB Function ==
  data: y input; dy output; dt input; tau input; ema_prev input; ema output
function [dy, ema] = realtime_derivative_ema(y, dt, tau, ema_prev)
    % Compute smoothed derivative using Exponential Moving Average
    %
    % Inputs:
    %   y        : Current measurement
    %   dt       : Time step
    %   tau      : Time constant for EMA filter (larger = more smoothing)
    %   ema_prev : Previous EMA value
    %
    % Outputs:
    %   dy  : Smoothed derivative estimate
    %   ema : Updated EMA value
    
    % Calculate smoothing factor from time constant
    alpha = 1 - exp(-dt ./ tau);
    
    % Update Exponential Moving Average
    ema = alpha .* y + (1 - alpha) .* ema_prev;
    
    % Compute derivative using finite difference on smoothed values
    dy = (ema - ema_prev) ./ dt;
end

== matlab function Experiment1/Simulate Plant Dynamics/BLUE Dynamics/Data @ Measurement Rate/Calculate True Time Step/MATLAB Function ==
  data: dt input; dt_out output; dataRate input
function dt_out = CheckforInvalidTime(dt, dataRate)

    if dt <= 0

        dt_out = dataRate;

    else

        dt_out = dt;

    end


end

== matlab function Experiment1/Thruster Control Code/Change BLUE Behavior/Calculate Duty Cycle/MATLAB Function5 ==
  data: H_final output; u_desired input; duty_cycles output; x0 input; thruster_dist2CG_RED parameter; F_red_X_nominal parameter; F_red_Y_nominal parameter; max_iters parameter; tol parameter
function [H_final, duty_cycles] = optimize_duty_cycle_with_decay( ...
    u_desired, x0, thruster_dist2CG_RED, F_red_X_nominal, F_red_Y_nominal, max_iters, tol)
    %OPTIMIZE_DUTY_CYCLE_WITH_DECAY 
    %   Iteratively optimizes thruster duty cycles while updating thrust decay.
    %
    %   Inputs:
    %       u_desired           - Desired force/torque vector [Fx; Fy; M] (3x1)
    %       x0                  - Initial guess for duty cycles (8x1)
    %       thruster_dist2CG_RED- Distances of thrusters from CG (vector, mm)
    %       F_red_X_nominal     - Nominal X-direction thruster force (scalar, N)
    %       F_red_Y_nominal     - Nominal Y-direction thruster force (scalar, N)
    %       max_iters           - Maximum optimization iterations
    %       tol                 - Convergence tolerance (on duty cycles)
    %
    %   Outputs:
    %       H_final     - Final H-matrix including thrust decay (3x8)
    %       duty_cycles - Optimized duty cycles (8x1)
    %

    % ---------------------------
    % Initialization
    % ---------------------------
    num_thrusters      = length(x0); %#ok<NASGU> % reserved if needed later
    duty_cycles        = x0;                     % current solution
    thrust_decay_factor = 1;                     % initial decay
    prev_duty_cycles   = duty_cycles + 2*tol;    % force first iteration

    % ---------------------------
    % Iterative optimization
    % ---------------------------
    for iter = 1:max_iters
        % Build system matrix H with current decay factor
        H = MakeHWithDecay(thruster_dist2CG_RED, F_red_X_nominal, ...
                           thrust_decay_factor, F_red_Y_nominal);

        % Solve constrained least squares (box constraints: 0 ≤ x ≤ 1)
        duty_cycles = custom_constrained_least_squares(H, u_desired, duty_cycles);

        % Update decay factor based on the current duty cycles
        [thrust_decay_factor, ~] = check_thrust_decay(duty_cycles);

        % Check convergence (∞-norm difference)
        if norm(duty_cycles - prev_duty_cycles, Inf) < tol
            H_final = MakeHWithDecayRecalculateForce(thruster_dist2CG_RED, ...
                        F_red_X_nominal, thrust_decay_factor, F_red_Y_nominal);
            return;
        end

        % Update reference for next iteration
        prev_duty_cycles = duty_cycles;
    end

    % If not converged within max_iters, return final H with last decay
    H_final = MakeHWithDecayRecalculateForce(thruster_dist2CG_RED, ...
                F_red_X_nominal, thrust_decay_factor, F_red_Y_nominal);
end


% ========================================================================
% Custom Constrained Least Squares Solver
% ========================================================================
function x_opt = custom_constrained_least_squares(H, b, x0)
    %CUSTOM_CONSTRAINED_LEAST_SQUARES
    %   Solves min_x ||H*x - b||^2 subject to 0 <= x <= 1
    %   using projected gradient descent with backtracking line search.
    %
    %   Inputs:
    %       H   - System matrix (3x8)
    %       b   - Desired vector (3x1)
    %       x0  - Initial guess (8x1)
    %
    %   Output:
    %       x_opt - Optimal duty cycle vector (8x1)

    % Parameters
    max_iterations = 100;
    tolerance      = 1e-6;
    alpha          = 0.01;  % initial step size
    beta           = 0.5;   % backtracking factor

    % Initialization
    x      = x0;
    x_prev = x0 + 2*tolerance;

    % Precompute matrices
    HtH = H' * H;
    Htb = H' * b;

    for iter = 1:max_iterations
        % Gradient of ||H*x - b||^2
        gradient = 2 * (HtH*x - Htb);

        % Store objective for comparison
        current_obj = norm(H*x - b)^2;

        % Backtracking line search
        step_size = alpha;
        for ls_iter = 1:20
            x_new = x - step_size * gradient;
            x_new = max(0, min(1, x_new)); % project into [0,1]

            new_obj = norm(H*x_new - b)^2;
            if new_obj < current_obj
                break; % accept step
            else
                step_size = step_size * beta;
            end
        end

        % Update
        x = x_new;

        % Convergence check
        if norm(x - x_prev) < tolerance
            break;
        end

        % Adaptive step size tuning
        if iter > 1 && new_obj < current_obj
            alpha = min(alpha * 1.1, 0.1); % speed up if progress
        else
            alpha = alpha * 0.9;           % slow down otherwise
        end

        % Store for next iteration
        x_prev = x;
    end

    x_opt = x;
end


% ========================================================================
% Construct H-matrix (with decay factor)
% ========================================================================
function H = MakeHWithDecay(thruster_dist2CG, F_X_nominal, thrust_decay_factor, F_Y_nominal)
    %MAKEHWITHDECAY
    %   Builds the H matrix that maps thruster duty cycles to [Fx; Fy; M],
    %   applying thrust decay.
    %
    %   Outputs H as (3x8)

    % Convert thruster arm distances to meters
    adjusted_dist = thruster_dist2CG / 1000;

    % Thruster directions (X, Y, and moment arm)
    Vec1 = [-1; -1;  0;  0;  1;  1;  0;  0]; % X
    Vec2 = [ 0;  0;  1;  1;  0;  0; -1; -1]; % Y
    Vec3 = adjusted_dist;                    % moment (Z)

    Mat1 = [Vec1, Vec2, Vec3]';

    % Thruster forces (scaled by decay)
    F_thrusters = [F_X_nominal; F_X_nominal; ...
                   F_Y_nominal; F_Y_nominal; ...
                   F_X_nominal; F_X_nominal; ...
                   F_Y_nominal; F_Y_nominal] * thrust_decay_factor;

    % Build diagonal scaling
    Mat2 = diag(F_thrusters / 2);

    % Final mapping
    H = Mat1 * Mat2;
end


% ========================================================================
% Construct H-matrix (recalculate full force with decay)
% ========================================================================
function H = MakeHWithDecayRecalculateForce(thruster_dist2CG, F_X_nominal, thrust_decay_factor, F_Y_nominal)
    %MAKEHWITHDECAYRECALCULATEFORCE
    %   Same as MakeHWithDecay but applies full nominal force scaling.

    adjusted_dist = thruster_dist2CG / 1000;

    Vec1 = [-1; -1;  0;  0;  1;  1;  0;  0];
    Vec2 = [ 0;  0;  1;  1;  0;  0; -1; -1];
    Vec3 = adjusted_dist;

    Mat1 = [Vec1, Vec2, Vec3]';

    F_thrusters = [F_X_nominal; F_X_nominal; ...
                   F_Y_nominal; F_Y_nominal; ...
                   F_X_nominal; F_X_nominal; ...
                   F_Y_nominal; F_Y_nominal] * thrust_decay_factor;

    Mat2 = diag(F_thrusters);

    H = Mat1 * Mat2;
end


% ========================================================================
% Thrust Decay Update Rule
% ========================================================================
function [thrust_decay_factor, count] = check_thrust_decay(PWMs)
    %CHECK_THRUST_DECAY
    %   Updates thrust decay factor based on average duty cycle.
    %
    %   Inputs:
    %       PWMs - Duty cycle vector (8x1)
    %
    %   Outputs:
    %       thrust_decay_factor - Adjusted decay factor (scalar)
    %       count               - Number of active thrusters

    % Normalize if needed
    if max(PWMs) > 1
        PWMs = PWMs / max(PWMs);
    end
    
    % Active thrusters
    count = sum(PWMs > 0);
    
    % Mean duty cycle (only active thrusters)
    avg_duty = sum(max(PWMs, 0)) / max(count, 1);
    
    % Update rule (piecewise)
    if avg_duty < 0.3 || count == 0
        thrust_decay_factor = 1;
    else
        thrust_decay_factor = max(0.6 - 2*avg_duty + 1, 0.5);
    end
end

== matlab function Experiment1/PhaseSpace Camera Code/Use Hardware to Obtain States/Store RED Data/Subsystem2/Enabled Subsystem/MATLAB Function ==
  data: y input; dy output; dt input; tau input; ema_prev input; ema output
function [dy, ema] = realtime_derivative_ema(y, dt, tau, ema_prev)
    % Compute smoothed derivative using Exponential Moving Average
    %
    % Inputs:
    %   y        : Current measurement
    %   dt       : Time step
    %   tau      : Time constant for EMA filter (larger = more smoothing)
    %   ema_prev : Previous EMA value
    %
    % Outputs:
    %   dy  : Smoothed derivative estimate
    %   ema : Updated EMA value
    
    % Calculate smoothing factor from time constant
    alpha = 1 - exp(-dt ./ tau);
    
    % Update Exponential Moving Average
    ema = alpha .* y + (1 - alpha) .* ema_prev;
    
    % Compute derivative using finite difference on smoothed values
    dy = (ema - ema_prev) ./ dt;
end

== matlab function Experiment1/PhaseSpace Camera Code/Use Hardware to Obtain States/Store BLACK Data/Calculate True Time Step/MATLAB Function ==
  data: dt input; dt_out output; dataRate input
function dt_out = CheckforInvalidTime(dt, dataRate)

    if dt <= 0

        dt_out = dataRate;

    else

        dt_out = dt;

    end


end

== matlab function Experiment1/PhaseSpace Camera Code/Use Hardware to Obtain States/Store RED Data/Calculate True Time Step/MATLAB Function ==
  data: dt input; dt_out output; dataRate input
function dt_out = CheckforInvalidTime(dt, dataRate)

    if dt <= 0

        dt_out = dataRate;

    else

        dt_out = dt;

    end


end

== matlab function Experiment1/PhaseSpace Camera Code/Use Hardware to Obtain States/Store BLACK Data/Subsystem1/Enabled Subsystem/MATLAB Function ==
  data: y input; dy output; dt input; tau input; ema_prev input; ema output
function [dy, ema] = realtime_derivative_ema(y, dt, tau, ema_prev)
    % Compute smoothed derivative using Exponential Moving Average
    %
    % Inputs:
    %   y        : Current measurement
    %   dt       : Time step
    %   tau      : Time constant for EMA filter (larger = more smoothing)
    %   ema_prev : Previous EMA value
    %
    % Outputs:
    %   dy  : Smoothed derivative estimate
    %   ema : Updated EMA value
    
    % Calculate smoothing factor from time constant
    alpha = 1 - exp(-dt ./ tau);
    
    % Update Exponential Moving Average
    ema = alpha .* y + (1 - alpha) .* ema_prev;
    
    % Compute derivative using finite difference on smoothed values
    dy = (ema - ema_prev) ./ dt;
end

== matlab function Experiment1/PhaseSpace Camera Code/Use Hardware to Obtain States/Store BLACK Data/Subsystem2/Enabled Subsystem/MATLAB Function ==
  data: y input; dy output; dt input; tau input; ema_prev input; ema output
function [dy, ema] = realtime_derivative_ema(y, dt, tau, ema_prev)
    % Compute smoothed derivative using Exponential Moving Average
    %
    % Inputs:
    %   y        : Current measurement
    %   dt       : Time step
    %   tau      : Time constant for EMA filter (larger = more smoothing)
    %   ema_prev : Previous EMA value
    %
    % Outputs:
    %   dy  : Smoothed derivative estimate
    %   ema : Updated EMA value
    
    % Calculate smoothing factor from time constant
    alpha = 1 - exp(-dt ./ tau);
    
    % Update Exponential Moving Average
    ema = alpha .* y + (1 - alpha) .* ema_prev;
    
    % Compute derivative using finite difference on smoothed values
    dy = (ema - ema_prev) ./ dt;
end

== matlab function Experiment1/PhaseSpace Camera Code/Use Hardware to Obtain States/Store BLUE Data/Calculate True Time Step/MATLAB Function ==
  data: dt input; dt_out output; dataRate input
function dt_out = CheckforInvalidTime(dt, dataRate)

    if dt <= 0

        dt_out = dataRate;

    else

        dt_out = dt;

    end


end

== matlab function Experiment1/PhaseSpace Camera Code/Use Hardware to Obtain States/Store BLUE Data/Subsystem1/Enabled Subsystem/MATLAB Function ==
  data: y input; dy output; dt input; tau input; ema_prev input; ema output
function [dy, ema] = realtime_derivative_ema(y, dt, tau, ema_prev)
    % Compute smoothed derivative using Exponential Moving Average
    %
    % Inputs:
    %   y        : Current measurement
    %   dt       : Time step
    %   tau      : Time constant for EMA filter (larger = more smoothing)
    %   ema_prev : Previous EMA value
    %
    % Outputs:
    %   dy  : Smoothed derivative estimate
    %   ema : Updated EMA value
    
    % Calculate smoothing factor from time constant
    alpha = 1 - exp(-dt ./ tau);
    
    % Update Exponential Moving Average
    ema = alpha .* y + (1 - alpha) .* ema_prev;
    
    % Compute derivative using finite difference on smoothed values
    dy = (ema - ema_prev) ./ dt;
end

== matlab function Experiment1/PhaseSpace Camera Code/Use Hardware to Obtain States/Store BLUE Data/Subsystem2/Enabled Subsystem/MATLAB Function ==
  data: y input; dy output; dt input; tau input; ema_prev input; ema output
function [dy, ema] = realtime_derivative_ema(y, dt, tau, ema_prev)
    % Compute smoothed derivative using Exponential Moving Average
    %
    % Inputs:
    %   y        : Current measurement
    %   dt       : Time step
    %   tau      : Time constant for EMA filter (larger = more smoothing)
    %   ema_prev : Previous EMA value
    %
    % Outputs:
    %   dy  : Smoothed derivative estimate
    %   ema : Updated EMA value
    
    % Calculate smoothing factor from time constant
    alpha = 1 - exp(-dt ./ tau);
    
    % Update Exponential Moving Average
    ema = alpha .* y + (1 - alpha) .* ema_prev;
    
    % Compute derivative using finite difference on smoothed values
    dy = (ema - ema_prev) ./ dt;
end
